simulink model "bldc_model_101119"  (R2018b)
settings: Solver=VariableStepAuto  StartTime=0.0  StopTime=10  RelTol=1e-3
values from neighbouring files (symbols this model uses):
  A = J*(Omega_phi + Omega)    [IMU.m]
  L = 0.42e-3    (= 0.00042)    [BLDC_simulator.m]    (also in engine_parameters.m; engine_parameters_20191210.m = 0.0005)
  phase = 6    [calculate_PWM.m]    (also in pwm_test.m)
libraries: powerlib x6, simulink_extras x1
settings Model: Creator=Paweł Tymiński  LastModifiedBy=Paweł Tymiński

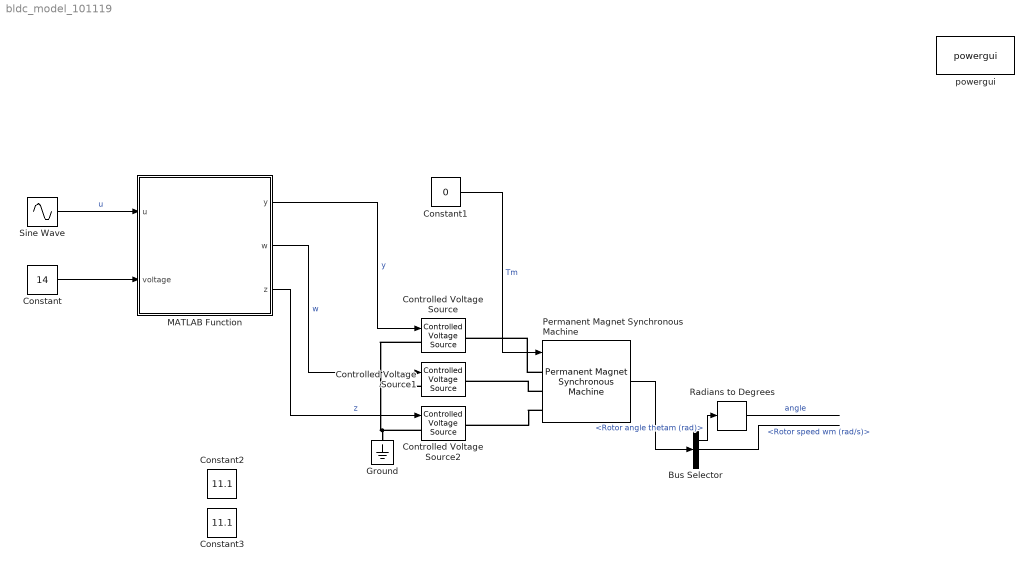
== system bldc_model_101119 ==
  Bus Selector : BusSelector  OutputSignals=Rotor angle thetam (rad),Rotor speed wm (rad/s),Electromagnetic torque Te (N*m)
  Constant : Constant  Value=14
  Constant1 : Constant  Value=0
  Constant2 : Constant  Value=11.1
  Constant3 : Constant  Value=11.1
  Controlled Voltage Source : powerlib/Electrical Sources/Controlled Voltage Source  Initialize=on  Source_Type=DC  Amplitude=0  Phase=0  Frequency=0  Measurements=None
  Controlled Voltage Source1 : powerlib/Electrical Sources/Controlled Voltage Source  Initialize=on  Source_Type=DC  Amplitude=0  Phase=0  Frequency=0  Measurements=None
  Controlled Voltage Source2 : powerlib/Electrical Sources/Controlled Voltage Source  Initialize=on  Source_Type=DC  Amplitude=0  Phase=0  Frequency=0  Measurements=None
  Ground : powerlib/Elements/Ground  LConnTagsString=a
  MATLAB Function : MATLAB Function  TreatAsAtomicUnit=on
  Permanent Magnet Synchronous Machine : powerlib/Machines/Permanent Magnet Synchronous Machine  NbPhases=3  FluxDistribution=Sinusoidal  RotorType=Round  MechanicalLoad=Torque Tm  PresetModel=No  ShowDetailedParameters=on  MeasurementBus=off  Resistance=6  Inductance=8.5e-3  dqInductances=[8.5e-3,8.5e-3]  La=0.006365  MachineConstant=Voltage Constant (V_peak L-L / krpm)  Flux=0.0052376  VoltageCst=13.3  TorqueCst=0.10999  Flat=120  Mechanical=[0.0001854 5.396e-05 14 0]  PolePairs=2  InitialConditions=[0,0, 0,0]  InitialConditions5ph=[0 0 0 0 0 0]  TsPowergui=0  TsBlock=-1  RefAngle=90 degrees behind phase A axis (modified Park)
      settings: SourceProductName=Simscape Power Systems
  Radians to Degrees : simulink_extras/Transformations/Radians to Degrees
  Sine Wave : Sin  Amplitude=300  Frequency=10  SampleTime=0
  powergui : powerlib/powergui  Priority=1  SimulationMode=Continuous  SampleTime=50e-6  frequency=60  Iterations=50  frequencyindice=0  Pbase=100e6  ErrMax=1e-4  UnitsV=kV  UnitsW=MW  buscounter=0  FunctionMessages=off  echomessages=off  EnableUseOfTLC=off  CurrentSourceSwitches=off  DisableSnubberDevices=off  DisableRonSwitches=off  DisableVfSwitches=off  DisplayEquations=off  SolverType=Tustin/Backward Euler (TBE)  Interpol=off  ExternalGateDelay=off  methode=off  Ts=100  x0status=blocks  SPID=on  SwTol=0  HookPort=off  RestoreLinks=warning  ResistiveCurrentMeasurement=off  Frange=[0:2:500]  Ylog=off  Xlog=on  ShowGrid=off  save=off  variable=ZData  structure=0  ZoomFFT=off  StartTime=0.0  cycles=1  DisplayStyle=1  fundamental=60  FreqAxis=off  MaxFrequency=1000  frequencyindicesteady=1  RmsSteady=1  display=off
  wires:
  Permanent Magnet Synchronous Machine/1 -> Bus Selector/1
  Radians to Degrees/1 -> ?  "angle"
  Bus Selector/2 -> ?  "<Rotor speed wm (rad/s)>"
  Constant/1 -> MATLAB Function/2(voltage)
  Sine Wave/1 -> MATLAB Function/1(u)  "u"
  MATLAB Function/1(y) -> Controlled Voltage Source/1  "y"
  MATLAB Function/2(w) -> Controlled Voltage Source1/1  "w"
  MATLAB Function/3(z) -> Controlled Voltage Source2/1  "z"
  Bus Selector/1 -> Radians to Degrees/1  "<Rotor angle thetam (rad)>"
  Constant1/1 -> Permanent Magnet Synchronous Machine/1  "Tm"
  connections:
  Permanent Magnet Synchronous Machine/LConn1 -- Controlled Voltage Source/RConn1
  Permanent Magnet Synchronous Machine/LConn3 -- Controlled Voltage Source2/RConn1
  Permanent Magnet Synchronous Machine/LConn2 -- Controlled Voltage Source1/RConn1
  Controlled Voltage Source2/LConn1 -- Controlled Voltage Source/LConn1 -- Controlled Voltage Source1/LConn1 -- Ground/LConn1

== matlab function bldc_model_101119/MATLAB Function ==
  data: u input; y output; voltage input; w output; z output

function[y,w,z] = calculate_PWM(u,voltage)
%konwersja kąta na wartości sygnału PWM do sterowania silnikiem BLDC
nop = 14;
phase=1;
PWM=0;
resolution = 2^12
; %rozdzielczość bitowa generowanego sygnału
    y=voltage;
    w=voltage;
    z=0;
%kalkulacja wartości PWM na poszczególne fazy

%konwersja kąta na wejściu na radiany
theta_error = u; %deg2rad(u);

%konwersja kąta mechanicznego na elektryczny (poślizg silnika)
theta_e = (theta_error*nop)/2;
%ograniczenie wartości kąta do wartości z zakresu 0-2 pi
theta_e = mod(theta_e,(2*pi));
if(theta_e < 0)
        theta_e = theta_e + (2*pi);
end

  if  theta_e <= 2/6*pi && theta_e>0
    PWM =round(resolution*(tan(theta_e)) /  (sin(2/3*pi)-cos(2/3*pi)*tan(theta_e)));
    phase=1;
elseif theta_e <= 4/6*pi && theta_e>2/6*pi
    PWM =round(resolution*-((tan(theta_e)*cos(2/3*pi)-sin(2/3*pi))/tan(theta_e)));
    phase=2;
elseif theta_e <= 6/6*pi && theta_e>4/6*pi
    PWM =round(resolution*(tan(theta_e)*cos(2/3*pi)-sin(2/3*pi)/sin(4/3*pi) -cos(4/3*pi)*tan(theta_e)));
    phase=3;
elseif theta_e <= 8/6*pi && theta_e>6/6*pi
    PWM =round(resolution*(tan(theta_e)*cos(4/3*pi)-sin(4/3*pi)/sin(2/3*pi) -cos(2/3*pi)*tan(theta_e)));
    phase=4;   
elseif theta_e <= 10/6*pi && theta_e>8/6*pi
    PWM =round(resolution*(sin(4/3*pi) - tan(theta_e)*cos(4/3*pi))/tan(theta_e));
    phase=5;
elseif theta_e <= 12/6*pi && theta_e>10/6*pi
    PWM =round(resolution*(tan(theta_e))/(sin(4/3*pi)-cos(4/3*pi)*tan(theta_e)));
    phase=6;
 end


if(phase==1)
    y=voltage;
    w=(voltage/resolution)*PWM;
    z=0;
elseif(phase==2)
    y=(voltage/resolution)*PWM;
    w=voltage;
    z=0;
elseif(phase==3)
    y=0;
    w=voltage;
    z=(voltage/resolution)*PWM;
elseif(phase==4)
    y=0;
    w=(voltage/resolution)*PWM;
    z=voltage;
elseif(phase==5)
    y=(voltage/resolution)*PWM;
    w=0;
    z=voltage;
else
    y=voltage;
    w=0;
    z=(voltage/resolution)*PWM;
end
end
